simulink model "convertidorBoost_2017a"  (R2017a)
settings: Solver=VariableStepAuto  StartTime=0.0  StopTime=20  RelTol=1e-3  EnableMultiTasking=on
values from neighbouring files (symbols this model uses):
  best = Xfin(3)    [Ag_estimar_Modelo_Convertidor_Boost.m]    (also in EvalConvertidorBoost.m = X(3))
  w0est = Xfin(1)    [Ag_estimar_Modelo_Convertidor_Boost.m]    (also in EvalConvertidorBoost.m = X(1))
  w1est = Xfin(2)    [Ag_estimar_Modelo_Convertidor_Boost.m]    (also in EvalConvertidorBoost.m = X(2))
settings Model: Creator=Jesús Lopez  LastModifiedBy=jesus
settings OptimizationCC: LifeSpan=inf
settings DebuggingCC: SFUnexpectedBacktrackingDiag=warning  SFNoUnconditionalDefaultTransitionDiag=warning  SFExecutionAtInitializationDiag=none
settings GRTTargetCC: TargetLangStandard=C89/C90 (ANSI)  GeneratePreprocessorConditionals=Disable all
settings ConfigComp: CovMetricSettings=dw  CovHtmlReporting=on  CovSaveCumulativeToWorkspaceVar=on  CovSaveSingleToWorkspaceVar=on  CovExternalEMLEnable=off

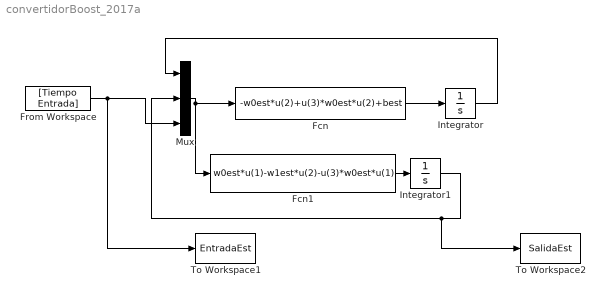
== system convertidorBoost_2017a ==
  Fcn : Fcn  Expr=-w0est*u(2)+u(3)*w0est*u(2)+best
  Fcn1 : Fcn  Expr=w0est*u(1)-w1est*u(2)-u(3)*w0est*u(1)
  From Workspace : FromWorkspace  VariableName=[Tiempo Entrada]  SampleTime=0.05
  Integrator : Integrator
  Integrator1 : Integrator
  Mux : Mux  Inputs=3
  To Workspace1 : ToWorkspace  VariableName=EntradaEst  SampleTime=0.05
  To Workspace2 : ToWorkspace  VariableName=SalidaEst  SampleTime=0.05
  wires:
  Mux/1 -> Fcn/1, Fcn1/1
  Fcn/1 -> Integrator/1
  Fcn1/1 -> Integrator1/1
  Integrator/1 -> Mux/1
  Integrator1/1 -> To Workspace2/1, Mux/2
  From Workspace/1 -> To Workspace1/1, Mux/3
